simulink model "HARDWARE (1)"  (R2023a)
settings: Solver=FixedStepDiscrete  StartTime=0.0  StopTime=10  FixedStep=0.001  RelTol=1e-3  EnableMultiTasking=on
undefined symbols (not defined in the file): HIL, K, kd_test, kp_test, P_start, Q, q1_ref_final, R, T, X_start
libraries: quarc_library x3, simulink x2
settings Model: Creator=leongold  LastModifiedBy=webb
settings SolverCC: PositivePriorityOrder=on
settings RTWCC: Description=QUARC Win64 Target Using Toolchain  SystemTargetFile=quarc_win64.tlc  Toolchain=QUARC win64 | nmake (64-bit Windows)  BuildConfiguration=Faster Runs
settings STFCustomTargetCC: SystemTargetFile=quarc_win64.tlc
settings GRTTargetCC: ParMdlRefBuildCompliant=off  CompOptLevelCompliant=off  CombineOutputUpdateFcns=off  MatFileLogging=off  CPPClassGenCompliant=off  GRTInterface=on  ExtMode=on  ExtModeMexFile=quarc_comm

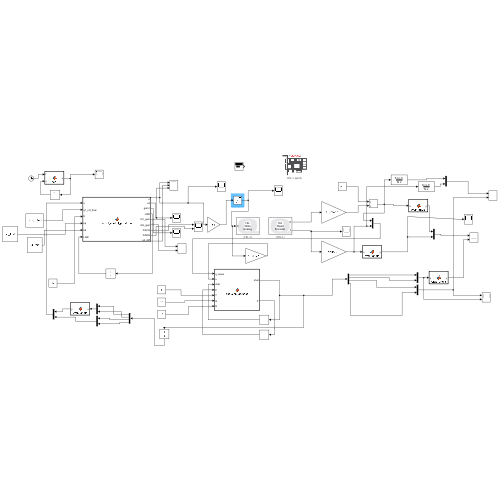
[thumbnail: Simulink's stored preview of the top-level diagram]
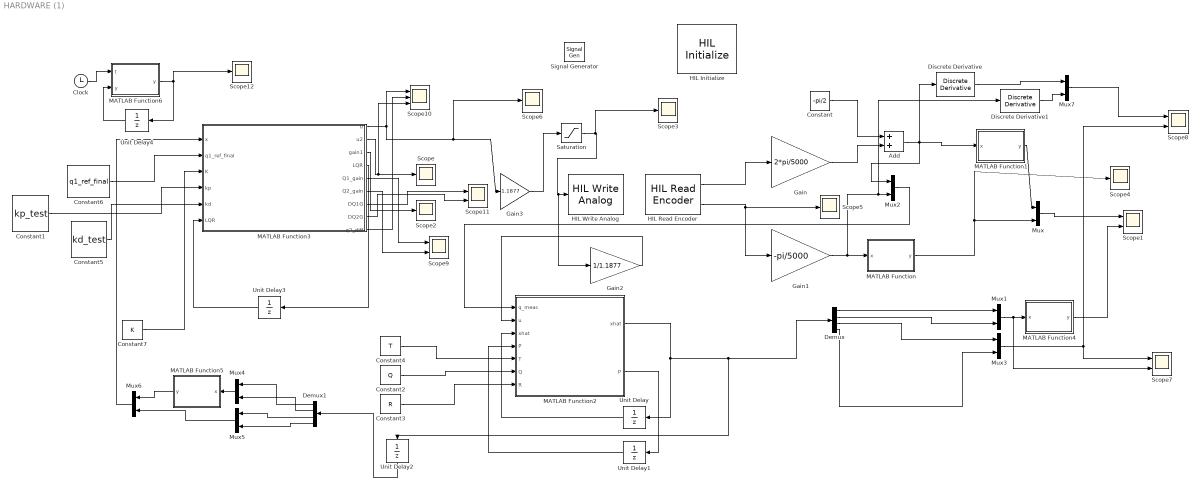
== system HARDWARE (1) ==
  Add : Sum
  Clock : Clock
  Constant : Constant  Value=-pi/2
  Constant1 : Constant  Value=kp_test
  Constant2 : Constant  Value=Q
  Constant3 : Constant  Value=R
  Constant4 : Constant  Value=T
  Constant5 : Constant  Value=kd_test
  Constant6 : Constant  Value=q1_ref_final
  Constant7 : Constant  Value=K
  Demux : Demux
  Demux1 : Demux
  Discrete Derivative : simulink/Discrete/Discrete Derivative  gainval=1.0  ICPrevScaledInput=0.0  OutMin=[]  OutMax=[]  OutDataType=fixdt(1, 16)  OutScaling=2^-10  DoSatur=off
  Discrete Derivative1 : simulink/Discrete/Discrete Derivative  gainval=1.0  ICPrevScaledInput=0.0  OutMin=[]  OutMax=[]  OutDataType=fixdt(1, 16)  OutScaling=2^-10  DoSatur=off
  Gain : Gain  Gain=2*pi/5000
  Gain1 : Gain  Gain=-pi/5000
  Gain2 : Gain  Gain=1/1.1877
  Gain3 : Gain  Gain=1.1877
  HIL Initialize : quarc_library/Data Acquisition/Generic/Configuration/HIL Initialize  object_name=HIL-1  board_type=q4  board_number=0  board_options=""  exclusive=off  active=on  hardware_clocks=[0:1]  clock_modes=[0 0]  initial_clock_frequencies=[]  set_clock_params_at_start=on  set_clock_params_at_switch_in=off  set_clock_frequencies_at_start=off  set_clock_frequencies_at_switch_in=off  analog_input_channels=[0:3]  analog_input_configurations=[]  analog_input_maximums=10  analog_input_minimums=-10  set_analog_input_params_at_start=off  set_analog_input_params_at_switch_in=off  analog_output_channels=[0:3]  analog_output_maximums=[10]  analog_output_minimums=[-10]  initial_analog_outputs=[0]  final_analog_outputs=[0]  watchdog_analog_outputs=0  set_analog_output_params_at_start=on  set_analog_output_params_at_switch_in=off  set_analog_outputs_at_start=on  set_analog_outputs_at_switch_in=off  set_analog_outputs_at_terminate=on  set_analog_outputs_at_switch_out=off  set_analog_outputs_on_watchdog=off  digital_input_channels=[]  digital_output_channels=[]  digital_output_configuration=[]  initial_digital_outputs=[1]  final_digital_outputs=[1]  watchdog_digital_outputs=[2]  set_digital_output_params_at_start=off  set_digital_output_params_at_switch_in=off  set_digital_outputs_at_start=on  set_digital_outputs_at_switch_in=off  set_digital_outputs_at_terminate=on  set_digital_outputs_at_switch_out=off  set_digital_outputs_on_watchdog=off  encoder_channels=[0:3]  quadrature=[4]  encoder_filter_frequency=(1/60e-9)/1  initial_encoder_counts=[0]  set_encoder_params_at_start=on  set_encoder_params_at_switch_in=off  set_encoder_counts_at_start=on  set_encoder_counts_at_switch_in=off  pwm_channels=[]  pwm_modes=[0]  pwm_frequency=(1/60e-9)/1024  pwm_configuration=[]  pwm_alignment=[]  pwm_polarity=[]  pwm_leading_deadband=[]  pwm_trailing_deadband=[]  initial_pwm_outputs=[0]  final_pwm_outputs=[0]  watchdog_pwm_outputs=[]  set_pwm_params_at_start=on  set_pwm_params_at_switch_in=off  set_pwm_outputs_at_start=on  set_pwm_outputs_at_switch_in=off  set_pwm_outputs_at_terminate=on  set_pwm_outputs_at_switch_out=off  set_pwm_outputs_on_watchdog=off  other_output_channels=[]  initial_other_outputs=[]  final_other_outputs=[]  watchdog_other_outputs=[]  set_other_outputs_at_start=off  set_other_outputs_at_switch_in=off  set_other_outputs_at_terminate=off  set_other_outputs_at_switch_out=off  set_other_outputs_on_watchdog=off
  HIL Read Encoder : quarc_library/Data Acquisition/Generic/Immediate I//O/HIL Read Encoder  object_name=HIL-1  channels=[0 1]  sample_time=qc_get_step_size  active=on  vector_output=off  data_type_mode=Inherit via back propagation  data_type=double
  HIL Write Analog : quarc_library/Data Acquisition/Generic/Immediate I//O/HIL Write Analog  object_name=HIL-1  channels=0  sample_time=-1  active=off  vector_input=off
  MATLAB Function : MATLAB Function  TreatAsAtomicUnit=on
  MATLAB Function1 : MATLAB Function  TreatAsAtomicUnit=on
  MATLAB Function2 : MATLAB Function  TreatAsAtomicUnit=on
  MATLAB Function3 : MATLAB Function  TreatAsAtomicUnit=on
  MATLAB Function4 : MATLAB Function  TreatAsAtomicUnit=on
  MATLAB Function5 : MATLAB Function  TreatAsAtomicUnit=on
  MATLAB Function6 : MATLAB Function  TreatAsAtomicUnit=on
  Mux{,1..7} (8 alike) : Mux  Inputs=2
  Saturation : Saturate  UpperLimit=6  LowerLimit=-6  LinearizeAsGain=off
  Scope{,2..6,12} (7 alike) : Scope
  Scope{1,7..9,11} (5 alike) : Scope  NumInputPorts=2
  Scope10 : Scope  NumInputPorts=3
  Signal Generator : SignalGenerator  Units=rad/sec
  Unit Delay : UnitDelay  InitialCondition=X_start  SampleTime=-1  HasFrameUpgradeWarning=on
  Unit Delay1 : UnitDelay  InitialCondition=P_start  SampleTime=-1  HasFrameUpgradeWarning=on
  Unit Delay2 : UnitDelay  InitialCondition=[-pi/2;0;0;0]  SampleTime=-1  HasFrameUpgradeWarning=on
  Unit Delay3 : UnitDelay  SampleTime=-1  HasFrameUpgradeWarning=on
  Unit Delay4 : UnitDelay  InitialCondition=kd_test  SampleTime=-1  HasFrameUpgradeWarning=on
  wires:
  HIL Read Encoder/1 -> Gain/1
  Gain/1 -> Add/2
  HIL Read Encoder/2 -> Scope5/1, Gain1/1
  Gain1/1 -> Discrete Derivative1/1, Mux2/2, MATLAB Function/1(x)
  MATLAB Function/1(y) -> Scope4/1, Mux/2
  MATLAB Function1/1(y) -> Mux/1
  Constant/1 -> Add/1
  Add/1 -> Discrete Derivative/1, Mux2/1, MATLAB Function1/1(x)
  Constant4/1 -> MATLAB Function2/5(T)
  Mux/1 -> Scope1/1
  Unit Delay/1 -> MATLAB Function2/3("xhat ")
  MATLAB Function2/2(P) -> Unit Delay1/1
  Unit Delay1/1 -> MATLAB Function2/4("P ")
  Constant2/1 -> MATLAB Function2/6(Q)
  Constant3/1 -> MATLAB Function2/7(R)
  Demux/1 -> Mux1/1
  Demux/2 -> Mux1/2
  Mux1/1 -> Scope7/2, MATLAB Function4/1(x)
  Constant1/1 -> MATLAB Function3/4(kp)
  Constant6/1 -> MATLAB Function3/2(q1_ref_final)
  MATLAB Function3/1(u) -> Gain3/1, Scope6/1, Scope10/1
  Saturation/1 -> Scope3/1, Gain2/1, HIL Write Analog/1
  MATLAB Function3/2(u2) -> Scope/1, Scope10/3
  Constant7/1 -> MATLAB Function3/3(K)
  Mux2/1 -> MATLAB Function2/1(q_meas)
  MATLAB Function4/1(y) -> Scope1/2
  Demux/3 -> Mux3/1
  Demux/4 -> Mux3/2
  Mux3/1 -> Scope7/1, Scope8/2
  MATLAB Function2/1(xhat) -> Unit Delay2/1, Demux/1, Unit Delay/1
  Demux1/1 -> Mux4/1
  Demux1/2 -> Mux4/2
  Demux1/3 -> Mux5/1
  Demux1/4 -> Mux5/2
  Mux4/1 -> MATLAB Function5/1(x)
  MATLAB Function5/1(y) -> Mux6/1
  Mux5/1 -> Mux6/2
  Mux6/1 -> MATLAB Function3/1(x)
  MATLAB Function3/3(gain1) -> Scope2/1
  Unit Delay2/1 -> Demux1/1
  Mux7/1 -> Scope8/1
  Discrete Derivative1/1 -> Mux7/2
  Discrete Derivative/1 -> Mux7/1
  MATLAB Function3/4(LQR) -> Unit Delay3/1
  Unit Delay3/1 -> MATLAB Function3/6("LQR ")
  MATLAB Function3/5(Q1_gain) -> Scope9/1
  MATLAB Function3/6(Q2_gain) -> Scope9/2
  MATLAB Function3/7(DQ1G) -> Scope11/1
  MATLAB Function3/8(DQ2G) -> Scope11/2
  Gain2/1 -> MATLAB Function2/2(u)
  MATLAB Function3/9(q2_diff) -> Scope10/2
  Gain3/1 -> Saturation/1
  Clock/1 -> MATLAB Function6/1(t)
  MATLAB Function6/1(y) -> Unit Delay4/1, Scope12/1
  Unit Delay4/1 -> MATLAB Function6/2("y ")
  Constant5/1 -> MATLAB Function3/5(kd)

== matlab function HARDWARE (1)/MATLAB Function1 ==
  data: x input; y output
function y = wrap_angle(x)

y = mod(x+pi, 2*pi) -pi;

== matlab function HARDWARE (1)/MATLAB Function ==
  data: x input; y output
function y = wrap_angle(x)

y = mod(x+pi, 2*pi) -pi;

== matlab function HARDWARE (1)/MATLAB Function2 ==
  data: q_meas input; u input; xhat output; xhat input; P input; T input; Q input; R input; P output
function [xhat, P] = ekf_step_acrobot(q_meas, u, xhat, P, T, Q, R)
% EKF for acrobot/pendubot-like system.
% State:       x = [q1; q2; dq1; dq2]
% Measurement: y = [q1; q2]
%
% Inputs:
%   q_meas : 2x1 measured angles [q1; q2]
%   u      : scalar input torque at this time step
%   xhat   : 4x1 prior state estimate at time k
%   P      : 4x4 prior covariance at time k
%   T      : sample time
%   p      : parameter struct for acrobot_dynamics
%   Q      : 4x4 process noise covariance (continuous-time-ish)
%   R      : 2x2 measurement noise covariance
%
% Outputs:
%   xhat   : 4x1 posterior state estimate at time k+1
%   P      : 4x4 posterior covariance at time k+1



    p.m1 = 1.0969;     % Mass of link 1 (kg)
    p.m2 = 0.8356;     % Mass of link 2 (kg)
    p.l1 = 0.1524;     % Length of link 1 (m)
    p.l2 = 0.2286;     % Length of link 2 (m)
    p.lc1 = 0.0754;    % Distance to center of mass of link 1 (m)
    p.lc2 = 0.0754;    % Distance to center of mass of link 2 (m)
    p.I1 = 0.0056;   % Moment of inertia of link 1 (kg·m^2)
    p.I2 = 0.0059;   % Moment of inertia of link 2 (kg·m^2)
    p.g = 9.81;     % Gravity (m/s^2)
    n = 4;
    I = eye(n);

    % ---------- 1) Prediction step (nonlinear) ----------
    % Use RK4 for better accuracy than simple Euler
    f = @(x) pendubot_dynamics(0, x, u, p);

    k1 = f(xhat);
    k2 = f(xhat + 0.5*T*k1);
    k3 = f(xhat + 0.5*T*k2);
    k4 = f(xhat + T*k3);

    x_pred = xhat + (T/6)*(k1 + 2*k2 + 2*k3 + k4);

    % Wrap angles to [-pi, pi] for numerical sanity
    

    % ---------- 2) Linearization at x_pred (Jacobian A) ----------
    A = numerical_jacobian_pendubot(@pendubot_dynamics, x_pred, u, p);

    % Discretize A and Q (simple approximation)
    Ad = I + A*T;
    Qd = Q * T;   % crude CT→DT mapping (often good enough if T small)

    % ---------- 3) Covariance prediction ----------
    P_pred = Ad * P * Ad' + Qd;

    % ---------- 4) Measurement model ----------
    % Measurement: y = [q1; q2] = h(x)
    % So h(x) = [x(1); x(2)], and C = dh/dx:
    C = [1 0 0 0;
         0 1 0 0];

    % Predicted measurement
    y_pred = [x_pred(1); x_pred(2)];

    % Innovation (wrap angle differences to handle 2*pi jumps)
    innov = [q_meas(1)-y_pred(1);
             q_meas(2)- y_pred(2)];

    % Innovation covariance
    S = C * P_pred * C' + R;

    % ---------- 5) Kalman gain ----------
    L = P_pred * C' / S;

    % ---------- 6) Update step ----------
    xhat = x_pred + L * innov;

    % Wrap angles again
   

    % Joseph form for covariance update (numerically robust)
    P = (I - L*C) * P_pred * (I - L*C)' + L * R * L';
end

== matlab function HARDWARE (1)/MATLAB Function3 ==
  data: x input; u output; q1_ref_final input; K input; kp input; kd input; u2 output; gain1 output; LQR input; LQR output; Q1_gain output; Q2_gain output; DQ1G output; DQ2G output; q2_diff output
function [u,u2,gain1, LQR, Q1_gain, Q2_gain, DQ1G, DQ2G, q2_diff] = hybrid_control_pendubot(x, q1_ref_final, K,kp, kd, LQR)
    q1  = x(1);  q2  = x(2);
    dq1 = x(3);  dq2 = x(4);
    q1_wrapped = mod(q1, 2*pi);
    q2_wrapped = abs(mod(q2, 2*pi));
    x_ref = [q1_ref_final; pi/2-q1_ref_final; 0; 0];
    dx = x-x_ref;
    Q2_correct = sign(q2) == -1*sign(dq2);
    in_LQR_region = abs(q1 - x_ref(1)) < 0.4 && abs(q2 -x_ref(2)) < 0.5 && abs(dq2) < 1.0 && Q2_correct;
    u2 = -(K(1)*dx(1) +K(2)*dx(2) +K(3)*dx(3)+K(4)*dx(4));
    Q1_gain = K(1)*dx(1);
    Q2_gain = K(2)*dx(2) ;
    DQ1G = K(3)*dx(3);
    DQ2G = K(4)*dx(4);
    m1 = 1.0969;     % Mass of link 1 (kg)
    m2 = 0.8356;     % Mass of link 2 (kg)
    l1 = 0.1524;     % Length of link 1 (m)
    l2 = 0.2286;     % Length of link 2 (m)
    lc1 = 0.0754;    % Distance to center of mass of link 1 (m)
    lc2 = 0.0754;    % Distance to center of mass of link 2 (m)
    I1 = 0.0056;   % Moment of inertia of link 1 (kg·m^2)
    I2 = 0.0059;   % Moment of inertia of link 2 (kg·m^2)
    g = 9.81;     % Gravity (m/s^2)

    d11 = m1*lc1^2 + m2*(l1^2 + lc2^2 + 2*l1*lc2*cos(q2)) + I1 + I2;
    d12 = m2*(lc2^2 + l1*lc2*cos(q2)) + I2;
    d21 = d12;
    d22 = m2*lc2^2 + I2;
    h1 = -m2*l1*lc2*sin(q2)*dq2^2 - 2*m2*l1*lc2*sin(q2)*dq1*dq2;
    h2 =  m2*l1*lc2*sin(q2)*dq1^2;
    phi1 = (m1*lc1 + m2*l1)*g*cos(q1) + m2*lc2*g*cos(q1 + q2);
    phi2 = m2*lc2*g*cos(q1 + q2);
    D1 =d11 -d12*d21/d22;
    H1 = h1 -d12*h2/d22;
    PHI1 = phi1 -d12*phi2/d22;
    
   
        
    v1 = kp * (q1_ref_final-q1) - kd * dq1;         % desired ddq1
        
    gain1 = q1_ref_final-q1;   
    u = D1*v1+PHI1+H1;
    if in_LQR_region || LQR ==1
        disp('LQR');
        u = u2;
        LQR =1;


    end
    q2_diff = abs(q2 -x_ref(2));
        % u = d21 * v1 + d22 * ddq2 + h2 + phi2;
   
    
end

== matlab function HARDWARE (1)/MATLAB Function4 ==
  data: x input; y output
function y = wrap_angle(x)

y = mod(x+pi, 2*pi) -pi;

== matlab function HARDWARE (1)/MATLAB Function5 ==
  data: x input; y output
function y = wrap_angle(x)

y = mod(x+pi, 2*pi) -pi;

== matlab function HARDWARE (1)/MATLAB Function6 ==
  data: t input; y output; y input
function y = fcn(t,y)
if mod(t,3) == 0 && t ~= 3
    y = y+0.1;
end
